simulink model "hybrid_ex_execution_order"  (R2017b)
settings: Solver=ode45  StartTime=0.0  StopTime=100  RelTol=1e-3  EnableMultiTasking=on
InitFcn:
  | P =0.6; I = 0.01; D = 0; b=20; m=1000;
settings Model: ExtModeTrigMode=oneshot  ExtModeArmWhenConnect=off  Creator=The MathWorks, Inc.  LastModifiedBy=ppolcz
settings DataIOCC: SaveFormat=Array  SignalLoggingName=logsOut
settings OptimizationCC: BlockReduction=off  BooleanDataType=off  ExpressionDepthLimit=2147483647  InitFltsAndDblsToZero=on  EfficientMapNaN2IntZero=off  LifeSpan=inf
settings DebuggingCC: AlgebraicLoopMsg=error  SaveWithParameterizedLinksMsg=none  UnderspecifiedInitializationDetection=Classic  MergeDetectMultiDrivingBlocksExec=none  CheckExecutionContextPreStartOutputMsg=on  CheckExecutionContextRuntimeOutputMsg=on  SignalResolutionControl=TryResolveAllWithWarning  BlockPriorityViolationMsg=error  MultiTaskDSMMsg=warning  MultiTaskCondExecSysMsg=none  FcnCallInpInsideContextMsg=warning  StateNameClashWarn=warning  StrictBusMsg=None  SFUnexpectedBacktrackingDiag=warning  SFNoUnconditionalDefaultTransitionDiag=warning  SFExecutionAtInitializationDiag=none
settings HardwareCC: ProdBitPerPointer=32  ProdBitPerSizeT=32  ProdBitPerPtrDiffT=32  ProdLargestAtomicFloat=None  ProdIntDivRoundTo=Undefined  ProdEndianess=Unspecified  ProdWordSize=32  ProdHWDeviceType=32-bit Generic  TargetUnknown=on
settings ModelReferenceCC: PropagateSignalLabelsOutOfModel=off
settings CodeAppCC: StateflowObjectComments=on
settings GRTTargetCC: TargetFcnLib=ansi_tfl_tmw.mat  TargetLangStandard=C89/C90 (ANSI)  GeneratePreprocessorConditionals=Disable all  CombineOutputUpdateFcns=off  GRTInterface=on
settings ConfigComp: CovMetricSettings=dw  CovHtmlReporting=on  CovSaveCumulativeToWorkspaceVar=on  CovSaveSingleToWorkspaceVar=on  CovExternalEMLEnable=off

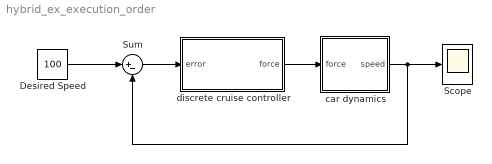
== system hybrid_ex_execution_order ==
  Desired Speed : Constant  Value=100
  Scope : Scope
  Sum : Sum  Inputs=|+-  SaturateOnIntegerOverflow=on  InputSameDT=on  OutDataTypeStr=Inherit: Same as first input
  car dynamics : Subsystem
  discrete cruise controller : Subsystem  TreatAsAtomicUnit=on
  wires:
  Sum/1 -> discrete cruise controller/1(error)
  car dynamics/1(speed) -> Scope/1, Sum/2
  discrete cruise controller/1(force) -> car dynamics/1(force)
  Desired Speed/1 -> Sum/1

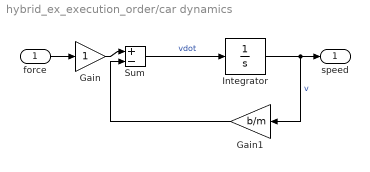
== system hybrid_ex_execution_order/car dynamics ==
  force : Inport
  Gain : Gain  Priority=2  SaturateOnIntegerOverflow=on  OutDataTypeStr=Inherit: Same as input  ParamDataTypeStr=Inherit: Same as input
  Gain1 : Gain  Priority=1  Gain=b/m  SaturateOnIntegerOverflow=on  OutDataTypeStr=Inherit: Same as input  ParamDataTypeStr=Inherit: Same as input
  Integrator : Integrator
  Sum : Sum  Inputs=|+-  SaturateOnIntegerOverflow=on  InputSameDT=on  OutDataTypeStr=Inherit: Same as first input
  speed : Outport
  wires:
  force/1 -> Gain/1
  Gain/1 -> Sum/1
  Gain1/1 -> Sum/2
  Integrator/1 -> speed/1, Gain1/1  "v"
  Sum/1 -> Integrator/1  "vdot"

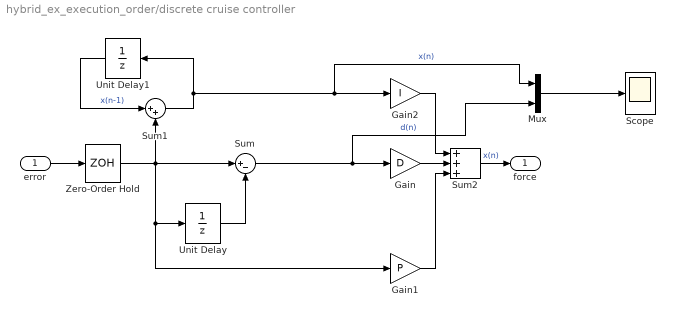
== system hybrid_ex_execution_order/discrete cruise controller ==
  error : Inport
  Gain : Gain  Priority=3  Gain=D  SaturateOnIntegerOverflow=on  OutDataTypeStr=Inherit: Same as input  ParamDataTypeStr=Inherit: Same as input
  Gain1 : Gain  Priority=2  Gain=P  SaturateOnIntegerOverflow=on  OutDataTypeStr=Inherit: Same as input  ParamDataTypeStr=Inherit: Same as input
  Gain2 : Gain  Priority=1  Gain=I  SaturateOnIntegerOverflow=on  OutDataTypeStr=Inherit: Same as input  ParamDataTypeStr=Inherit: Same as input
  Mux : Mux  Inputs=2
  Scope : Scope
  Sum : Sum  Inputs=|+-  SaturateOnIntegerOverflow=on  InputSameDT=on  OutDataTypeStr=Inherit: Same as first input
  Sum1 : Sum  Inputs=|++  SaturateOnIntegerOverflow=on  InputSameDT=on  OutDataTypeStr=Inherit: Same as first input
  Sum2 : Sum  Inputs=+++  SaturateOnIntegerOverflow=on  InputSameDT=on  OutDataTypeStr=Inherit: Same as first input
  Unit Delay : UnitDelay  SampleTime=.02
  Unit Delay1 : UnitDelay  SampleTime=.02
  Zero-Order Hold : ZeroOrderHold  SampleTime=.02
  force : Outport
  wires:
  Sum2/1 -> force/1  "x(n)"
  Gain1/1 -> Sum2/3
  Gain/1 -> Sum2/2
  Gain2/1 -> Sum2/1
  Sum/1 -> Mux/2, Gain/1  "d(n)"
  Sum1/1 -> Unit Delay1/1, Mux/1, Gain2/1  "x(n)"
  Unit Delay1/1 -> Sum1/1  "x(n-1)"
  Unit Delay/1 -> Sum/2
  Zero-Order Hold/1 -> Sum1/2, Gain1/1, Unit Delay/1, Sum/1
  error/1 -> Zero-Order Hold/1
  Mux/1 -> Scope/1
